simulink model "Sim_Plant"  (R2020b)
settings: Solver=ode3  StartTime=0.0  StopTime=10  FixedStep=0.01  RelTol=1e-3
values from neighbouring files (symbols this model uses):
  B = [0 0 13.9 13.7]'    [Initialize_NonLinear.m]
  K = K_Report    [Initialize_NonLinear.m]    (also in ResultSaver.m = K_LQR_new)
undefined symbols (not defined in the file or in its folder): A, C, gaussian
libraries: simulink x1
settings Model: Creator=Amir  LastModifiedBy=vahed

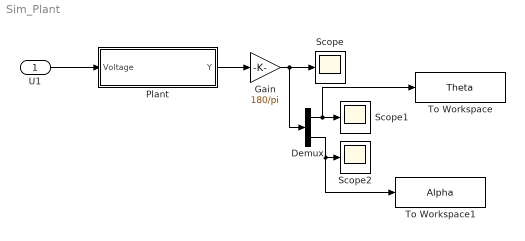
== system Sim_Plant ==
  U1 : Inport
  Demux : Demux  Outputs=2
  Gain : Gain  Gain=180/pi
  Plant : Subsystem
  Scope : Scope
  Scope1 : Scope
  Scope2 : Scope
  To Workspace : ToWorkspace  VariableName=Theta  SaveFormat=Timeseries  SampleTime=-1
  To Workspace1 : ToWorkspace  VariableName=Alpha  SaveFormat=Timeseries  SampleTime=-1
  wires:
  U1/1 -> Plant/1(Voltage)
  Plant/1(Y) -> Gain/1
  Gain/1 -> Demux/1, Scope/1
  Demux/1 -> To Workspace/1, Scope1/1
  Demux/2 -> To Workspace1/1, Scope2/1

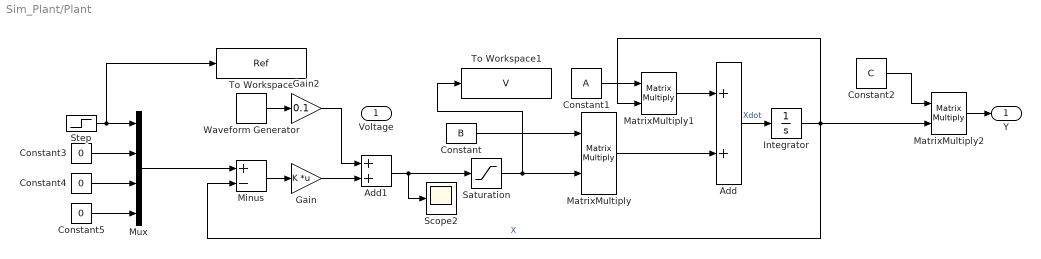
== system Sim_Plant/Plant ==
  Voltage : Inport
  Add : Sum
  Add1 : Sum
  Constant : Constant  Value=B
  Constant1 : Constant  Value=A
  Constant2 : Constant  Value=C
  Constant3 : Constant  Value=0
  Constant4 : Constant  Value=0
  Constant5 : Constant  Value=0
  Gain : Gain  Gain=K  Multiplication=Matrix(K*u)
  Gain2 : Gain  Gain=0.1
  Integrator : Integrator  InitialCondition=[0 0 0 0]
  MatrixMultiply : Product  Multiplication=Matrix(*)
  MatrixMultiply1 : Product  Multiplication=Matrix(*)
  MatrixMultiply2 : Product  Multiplication=Matrix(*)
  Minus : Sum  Inputs=+-
  Mux : Mux
  Saturation : Saturate  UpperLimit=15  LowerLimit=-15
  Scope2 : Scope
  Step : Step  Time=2  After=pi/2  SampleTime=0
  To Workspace : ToWorkspace  VariableName=Ref  SaveFormat=Timeseries  SampleTime=-1
  To Workspace1 : ToWorkspace  VariableName=V  SaveFormat=Timeseries  SampleTime=-1
  Waveform Generator : simulink/Sources/Waveform Generator  OutMin=[]  OutMax=[]  OutDataTypeStr=double  SelectedSignal=1  Signals=gaussian('Mean',0,'Variance',1)  BlockNames=MultiportSwitch_429da8b632dd481  SampleTime=0.01
  Y : Outport
  wires:
  Constant/1 -> MatrixMultiply/1
  MatrixMultiply/1 -> Add/2
  Add/1 -> Integrator/1  "Xdot"
  MatrixMultiply1/1 -> Add/1
  MatrixMultiply2/1 -> Y/1
  Constant2/1 -> MatrixMultiply2/1
  Constant1/1 -> MatrixMultiply1/1
  Step/1 -> To Workspace/1, Mux/1
  Constant3/1 -> Mux/2
  Constant4/1 -> Mux/3
  Constant5/1 -> Mux/4
  Mux/1 -> Minus/1
  Minus/1 -> Gain/1
  Waveform Generator/1 -> Gain2/1
  Gain2/1 -> Add1/1
  Gain/1 -> Add1/2
  Add1/1 -> Saturation/1, Scope2/1
  Integrator/1 -> Minus/2, MatrixMultiply2/2, MatrixMultiply1/2  "X"
  Saturation/1 -> MatrixMultiply/2, To Workspace1/1
